simulink model "simulation_rocket"  (R2018a)
settings: Solver=FixedStepAuto  StartTime=0.0  StopTime=200  RelTol=1e-3
undefined symbols (not defined in the file): A_nozzle, area, C_A_0, C_A_Alpha, C_A_Beta, C_Mpitch_alpha, C_Mpitch_q, C_Mroll_0, C_Mroll_p, C_Myaw_beta, C_Myaw_r, C_N_0, C_N_Alpha, C_S_0, C_S_Beta, dot_m, Earth, engine_number, J, l, LF, m, omega_E, omega_J, p_exit, r_gimble, r_init, rotationZ, serial, t_burn, v_exit, WGS84
libraries: aerolibtransform2 x3, aerolibutil x3, instrumentlib x2, aerolibatmos2 x1, aerolibgravity2 x1, sharedutil x1, simulink_extras x1
settings Model: PacingRate=5  ExtModeTrigDuration=2  Creator=hrist  LastModifiedBy=hrist
settings DataIOCC: ExternalInput=[0 0 0 0 0 0]  InitialState=[]  LoadInitialState=on  SaveFormat=StructureWithTime
settings OptimizationCC: EnhancedBackFolding=on  PassReuseOutputArgsAs=Individual arguments  MaxStackSize=64  OptimizeBlockOrder=speed  DifferentSizesBufferReuse=on  OptimizationCustomize=off
settings DebuggingCC: ParameterTunabilityLossMsg=error
settings HardwareCC: ProdBitPerInt=16  ProdBitPerPointer=16  ProdBitPerSizeT=16  ProdBitPerPtrDiffT=16  ProdLargestAtomicFloat=None  ProdWordSize=8  ProdHWDeviceType=Atmel->AVR
settings ModelReferenceCC: PropagateSignalLabelsOutOfModel=off
settings SFSimCC: MATLABDynamicMemAlloc=off
settings RTWCC: SystemTargetFile=ert.tlc  HardwareBoard=Arduino Uno  TLCOptions=-aInlineSetEventsForThisBaseRateFcn=TLC_FALSE -aSuppressMultiTaskScheduler=TLC_FALSE -aRateBasedStepFcn=1  TemplateMakefile=ert_default_tmf  GenerateReport=on  Toolchain=Arduino AVR  BuildConfiguration=Faster Runs  IncludeHyperlinkInReport=on  LaunchReport=on  GenerateTraceInfo=on  GenerateTraceReport=on  GenerateTraceReportSl=on  GenerateTraceReportSf=on  GenerateTraceReportEml=on
settings CodeAppCC: ForceParamTrailComments=on  IgnoreCustomStorageClasses=off  OperatorAnnotations=on  SimulinkDataObjDesc=on  SFDataObjDesc=on  InsertBlockDesc=on
settings ERTTargetCC: SupportContinuousTime=on  SupportVariableSizeSignals=on

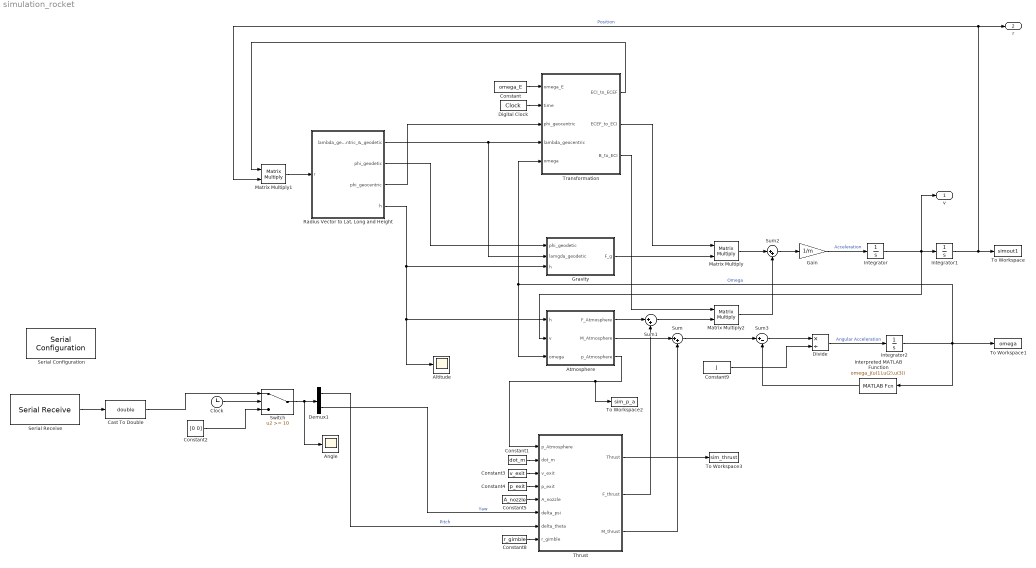
== system simulation_rocket ==
  "Altitude " : Scope
  Angle : Scope
  Atmosphere : Subsystem
  Cast To Double : DataTypeConversion  OutDataTypeStr=double
  Clock : Clock
  Constant : Constant  Value=omega_E
  Constant1 : Constant  Value=dot_m
  Constant2 : Constant  Value=[0 0]  VectorParams1D=off
  Constant3 : Constant  Value=v_exit
  Constant4 : Constant  Value=p_exit
  Constant5 : Constant  Value=A_nozzle
  Constant8 : Constant  Value=r_gimble
  Constant9 : Constant  Value=J  VectorParams1D=off
  Demux1 : Demux  Outputs=2
  Digital Clock : DigitalClock
  Divide : Product  Inputs=*/
  Gain : Gain  Gain=1/m
  Gravity : Subsystem
  Integrator : Integrator  InitialCondition=[600 0 0]
  Integrator1 : Integrator  InitialCondition=r_init
  Integrator2 : Integrator  InitialCondition=[0; 0; 0]
  Interpreted MATLAB Function : MATLABFcn  MATLABFcn=omega_J(u(1),u(2),u(3))
  Matrix Multiply : Product  Multiplication=Matrix(*)
  Matrix Multiply1 : Product  Multiplication=Matrix(*)
  Matrix Multiply2 : Product  Multiplication=Matrix(*)
  "Radius Vector to Lat, Long and Height " : Subsystem
  Serial Configuration : instrumentlib/Serial Configuration  Priority=-200000  ComPortMenu=<Please select a port...>  ComPort=COM6  ObjConstructor=serial('COM6');  BaudRate=115200  DataBits=8  Parity=none  StopBits=1  FlowControl=none  Timeout=10  ByteOrder=LittleEndian
  Serial Receive : instrumentlib/Serial Receive  ComPortMenu=<Please select a port...>  ComPort=COM6  ObjConstructor=serial('COM6');  Header=A  Terminator=LF ('\n')  DataSize="[1  2]"  DataType=single  EnableBlockingMode=on  ActionDataUnavailable=Output last received value  CustomValue=0  SampleTime=0.05
  Sum : Sum  Inputs=|++
  Sum1 : Sum  Inputs=|++
  Sum2 : Sum  Inputs=|++
  Sum3 : Sum  Inputs=|+-
  Switch : Switch  Threshold=10
  Thrust : Subsystem
  To Workspace : ToWorkspace  VariableName=simout1  SaveFormat=Timeseries  SampleTime=-1
  To Workspace1 : ToWorkspace  VariableName=omega  SampleTime=-1
  To Workspace2 : ToWorkspace  VariableName=sim_p_a  SaveFormat=Structure With Time  SampleTime=-1
  To Workspace3 : ToWorkspace  VariableName=sim_thrust  SaveFormat=Structure With Time  SampleTime=-1
  "Transformation " : Subsystem
  v : Outport
  r : Outport  Port=2
  wires:
  Constant/1 -> "Transformation "/1("omega_E ")
  Digital Clock/1 -> "Transformation "/2(time)
  "Radius Vector to Lat, Long and Height "/1("lambda_geocentric_&_geodetic ") -> Gravity/2(lamgda_geodetic), "Transformation "/4(lambda_geocentric)
  "Radius Vector to Lat, Long and Height "/2(phi_geodetic) -> Gravity/1(phi_geodetic)
  "Radius Vector to Lat, Long and Height "/4(h) -> "Altitude "/1, Atmosphere/1(h), Gravity/3(h)
  Atmosphere/3(p_Atmosphere) -> To Workspace2/1, Thrust/1(p_Atmosphere)
  Constant1/1 -> Thrust/2(dot_m)
  Constant3/1 -> Thrust/3(v_exit)
  Constant4/1 -> Thrust/4(p_exit)
  Constant5/1 -> Thrust/5(A_nozzle)
  Constant8/1 -> Thrust/8(r_gimble)
  Atmosphere/2(M_Atmosphere) -> Sum/1
  Thrust/3(M_thrust) -> Sum/2
  Gravity/1(F_g) -> Matrix Multiply/2
  "Transformation "/2(ECEF_to_ECI) -> Matrix Multiply/1
  Atmosphere/1("F_Atmosphere ") -> Sum1/1
  Thrust/2(F_thrust) -> Sum1/2
  Sum1/1 -> Matrix Multiply2/2
  "Transformation "/3(B_to_ECI) -> Matrix Multiply2/1
  Matrix Multiply/1 -> Sum2/1
  Matrix Multiply2/1 -> Sum2/2
  Sum2/1 -> Gain/1
  Gain/1 -> Integrator/1  "Acceleration"
  Integrator1/1 -> r/1, Matrix Multiply1/2, To Workspace/1  "Position"
  Sum/1 -> Sum3/1
  Sum3/1 -> Divide/1
  Constant9/1 -> Divide/2
  Divide/1 -> Integrator2/1  "Angular Acceleration"
  Integrator2/1 -> Interpreted MATLAB Function/1, To Workspace1/1, Atmosphere/3(omega), "Transformation "/5(omega)  "Omega"
  Interpreted MATLAB Function/1 -> Sum3/2
  "Radius Vector to Lat, Long and Height "/3(phi_geocentric) -> "Transformation "/3(phi_geocentric)
  "Transformation "/1(ECI_to_ECEF) -> Matrix Multiply1/1
  Matrix Multiply1/1 -> "Radius Vector to Lat, Long and Height "/1("r ")
  Integrator/1 -> Atmosphere/2(v), v/1, Integrator1/1
  Thrust/1(Thrust) -> To Workspace3/1
  Demux1/1 -> Thrust/7(delta_theta)  "Pitch"
  Demux1/2 -> Thrust/6(delta_psi)  "Yaw"
  Serial Receive/1 -> Cast To Double/1
  Switch/1 -> Angle/1, Demux1/1
  Clock/1 -> Switch/2
  Constant2/1 -> Switch/3
  Cast To Double/1 -> Switch/1

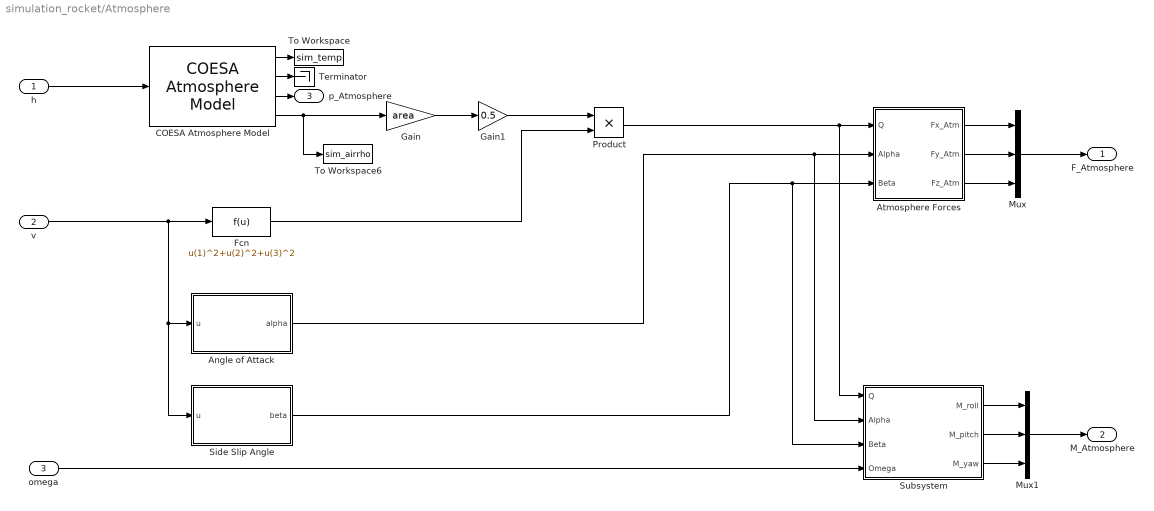
== system simulation_rocket/Atmosphere ==
  h : Inport
  v : Inport  Port=2
  omega : Inport  Port=3
  Angle of Attack : MATLAB Function  TreatAsAtomicUnit=on
  Atmosphere Forces : Subsystem
  COESA Atmosphere Model : aerolibatmos2/COESA Atmosphere Model  units=Metric (MKS)  spec=1976 COESA-extended U.S. Standard Atmosphere  model=Profile  profile_var=High temperature  profile_percent=1%  profile_alt=5 km (16404 ft)  envelope_var=High temperature  envelope_percent=1%  action=Warning
  Fcn : Fcn  Expr=u(1)^2+u(2)^2+u(3)^2
  Gain : Gain  Gain=area
  Gain1 : Gain  Gain=0.5
  Mux : Mux  Inputs=3
  Mux1 : Mux  Inputs=3
  Product : Product
  Side Slip Angle : MATLAB Function  TreatAsAtomicUnit=on
  Subsystem : Subsystem
  Terminator : Terminator
  To Workspace : ToWorkspace  VariableName=sim_temp  SaveFormat=Structure With Time  SampleTime=-1
  To Workspace6 : ToWorkspace  VariableName=sim_airrho  SaveFormat=Structure With Time  SampleTime=-1
  "F_Atmosphere " : Outport
  M_Atmosphere : Outport  Port=2
  p_Atmosphere : Outport  Port=3
  wires:
  COESA Atmosphere Model/2 -> Terminator/1
  h/1 -> COESA Atmosphere Model/1
  v/1 -> Side Slip Angle/1(u), Angle of Attack/1(u), Fcn/1
  COESA Atmosphere Model/4 -> To Workspace6/1, Gain/1
  Gain/1 -> Gain1/1
  Gain1/1 -> Product/1
  Angle of Attack/1(alpha) -> Subsystem/2(Alpha), Atmosphere Forces/2(Alpha)
  Side Slip Angle/1(beta) -> Subsystem/3(Beta), Atmosphere Forces/3(Beta)
  Atmosphere Forces/3(Fz_Atm) -> Mux/3
  Atmosphere Forces/2(Fy_Atm) -> Mux/2
  Atmosphere Forces/1("Fx_Atm ") -> Mux/1
  Mux/1 -> "F_Atmosphere "/1
  Fcn/1 -> Product/2
  omega/1 -> Subsystem/4(Omega)
  Product/1 -> Subsystem/1(Q), Atmosphere Forces/1(Q)
  Subsystem/1(M_roll) -> Mux1/1
  Subsystem/2(M_pitch) -> Mux1/2
  Subsystem/3(M_yaw) -> Mux1/3
  Mux1/1 -> M_Atmosphere/1
  COESA Atmosphere Model/3 -> p_Atmosphere/1
  COESA Atmosphere Model/1 -> To Workspace/1

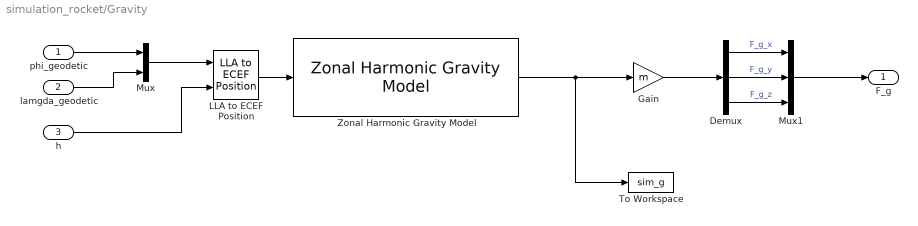
== system simulation_rocket/Gravity ==
  phi_geodetic : Inport
  lamgda_geodetic : Inport  Port=2
  h : Inport  Port=3
  Demux : Demux  Outputs=3
  Gain : Gain  Gain=m
  LLA to ECEF Position : aerolibtransform2/LLA to ECEF Position  units=Metric (MKS)  ptype=Earth (WGS84)  F=1/298.257223563  R=6378137
      settings: SourceProductName=Aerospace Blockset  SourceProductBaseCode=AE
  Mux : Mux  Inputs=2
  Mux1 : Mux  Inputs=3
  To Workspace : ToWorkspace  VariableName=sim_g  SaveFormat=Structure With Time  SampleTime=-1
  Zonal Harmonic Gravity Model : aerolibgravity2/Zonal Harmonic Gravity Model  units=Metric (MKS)  degree=4  action=Warning  ptype=Earth  R=6378136.3  GM=398600441500000  jvalue=[1.0826269e-03 -2.5323000e-06 -1.6204000e-06]
      settings: SourceProductName=Aerospace Blockset  SourceProductBaseCode=AE
  F_g : Outport
  wires:
  LLA to ECEF Position/1 -> Zonal Harmonic Gravity Model/1
  h/1 -> LLA to ECEF Position/2
  Mux/1 -> LLA to ECEF Position/1
  phi_geodetic/1 -> Mux/1
  lamgda_geodetic/1 -> Mux/2
  Zonal Harmonic Gravity Model/1 -> To Workspace/1, Gain/1
  Gain/1 -> Demux/1
  Demux/1 -> Mux1/1  "F_g_x"
  Demux/2 -> Mux1/2  "F_g_y"
  Demux/3 -> Mux1/3  "F_g_z"
  Mux1/1 -> F_g/1

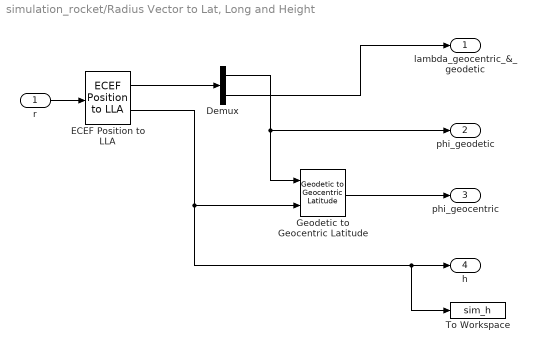
== system simulation_rocket/Radius Vector to Lat, Long and Height  ==
  "r " : Inport
  Demux : Demux  Outputs=2
  ECEF Position to LLA : aerolibtransform2/ECEF Position to LLA  units=Metric (MKS)  ptype=Earth (WGS84)  F=1/298.257223563  R=6378137
      settings: SourceProductName=Aerospace Blockset  SourceProductBaseCode=AE
  Geodetic to Geocentric Latitude : aerolibtransform2/Geodetic to  Geocentric Latitude  units=Metric (MKS)  ptype=Earth (WGS84)  F=1/298.257223563  R=6378137  wraplatitude=on
      settings: SourceProductName=Aerospace Blockset  SourceProductBaseCode=AE
  To Workspace : ToWorkspace  VariableName=sim_h  SaveFormat=Structure With Time  SampleTime=-1
  "lambda_geocentric_&_geodetic " : Outport
  phi_geodetic : Outport  Port=2
  phi_geocentric : Outport  Port=3
  h : Outport  Port=4
  wires:
  "r "/1 -> ECEF Position to LLA/1
  ECEF Position to LLA/1 -> Demux/1
  ECEF Position to LLA/2 -> To Workspace/1, h/1, Geodetic to Geocentric Latitude/2
  Demux/1 -> phi_geodetic/1, Geodetic to Geocentric Latitude/1
  Demux/2 -> "lambda_geocentric_&_geodetic "/1
  Geodetic to Geocentric Latitude/1 -> phi_geocentric/1

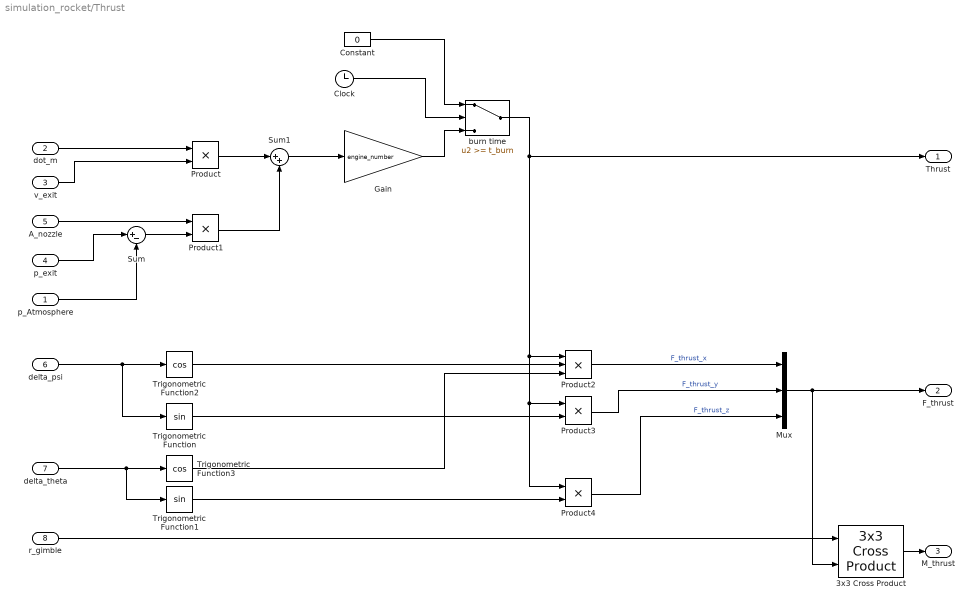
== system simulation_rocket/Thrust ==
  p_Atmosphere : Inport
  dot_m : Inport  Port=2
  v_exit : Inport  Port=3
  p_exit : Inport  Port=4
  A_nozzle : Inport  Port=5
  delta_psi : Inport  Port=6
  delta_theta : Inport  Port=7
  r_gimble : Inport  Port=8
  3x3 Cross Product : sharedutil/3x3 Cross Product  aMode=aMode
      settings: SourceProductBaseCode=AE
  Clock : Clock
  Constant : Constant  Value=0
  Gain : Gain  Gain=engine_number
  Mux : Mux  Inputs=3
  Product{,1,3..4} (4 alike) : Product
  Product2 : Product  Inputs=3
  Sum : Sum  Inputs=|+-
  Sum1 : Sum  Inputs=|++
  Trigonometric Function : Trigonometry
  Trigonometric Function1 : Trigonometry
  Trigonometric Function2 : Trigonometry  Operator=cos
  Trigonometric Function3 : Trigonometry  Operator=cos
  burn time : Switch  Threshold=t_burn
  Thrust : Outport
  F_thrust : Outport  Port=2
  M_thrust : Outport  Port=3
  wires:
  dot_m/1 -> Product/1
  v_exit/1 -> Product/2
  A_nozzle/1 -> Product1/1
  Sum/1 -> Product1/2
  p_exit/1 -> Sum/1
  p_Atmosphere/1 -> Sum/2
  Product/1 -> Sum1/1
  Product1/1 -> Sum1/2
  Sum1/1 -> Gain/1
  delta_psi/1 -> Trigonometric Function/1, Trigonometric Function2/1
  delta_theta/1 -> Trigonometric Function1/1, Trigonometric Function3/1
  Trigonometric Function2/1 -> Product2/2
  Trigonometric Function3/1 -> Product2/3
  Trigonometric Function/1 -> Product3/2
  Trigonometric Function1/1 -> Product4/2
  Product2/1 -> Mux/1  "F_thrust_x"
  Product3/1 -> Mux/2  "F_thrust_y"
  Product4/1 -> Mux/3  "F_thrust_z"
  Mux/1 -> 3x3 Cross Product/2, F_thrust/1
  r_gimble/1 -> 3x3 Cross Product/1
  3x3 Cross Product/1 -> M_thrust/1
  burn time/1 -> Thrust/1, Product4/1, Product3/1, Product2/1
  Constant/1 -> burn time/1
  Clock/1 -> burn time/2
  Gain/1 -> burn time/3

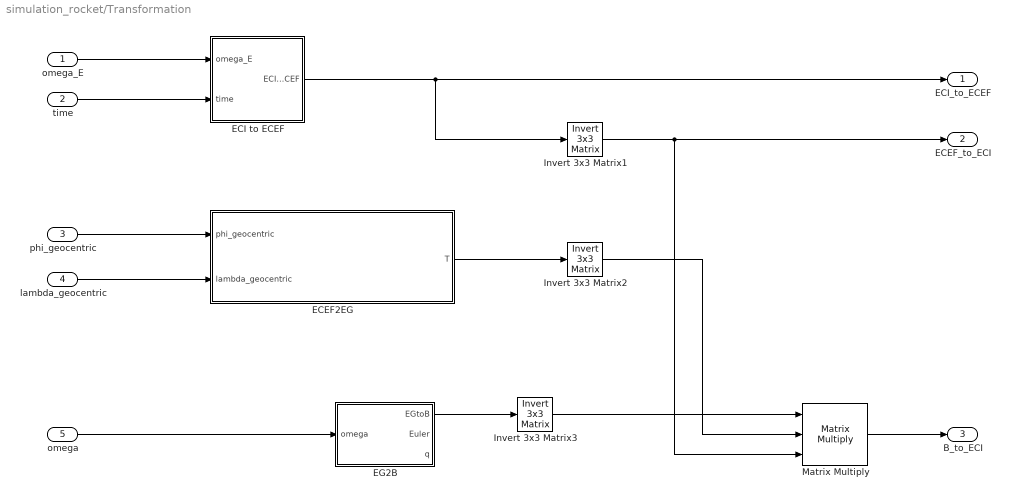
== system simulation_rocket/Transformation  ==
  "omega_E " : Inport
  time : Inport  Port=2
  phi_geocentric : Inport  Port=3
  lambda_geocentric : Inport  Port=4
  omega : Inport  Port=5
  ECEF2EG : MATLAB Function  TreatAsAtomicUnit=on
  ECI to ECEF : Subsystem
  EG2B : Subsystem
  Invert 3x3 Matrix1 : aerolibutil/Invert  3x3 Matrix
  Invert 3x3 Matrix2 : aerolibutil/Invert  3x3 Matrix
  Invert 3x3 Matrix3 : aerolibutil/Invert  3x3 Matrix
  Matrix Multiply : Product  Inputs=3  Multiplication=Matrix(*)
  ECI_to_ECEF : Outport
  ECEF_to_ECI : Outport  Port=2
  B_to_ECI : Outport  Port=3
  wires:
  "omega_E "/1 -> ECI to ECEF/1(omega_E)
  time/1 -> ECI to ECEF/2(time)
  phi_geocentric/1 -> ECEF2EG/1(phi_geocentric)
  lambda_geocentric/1 -> ECEF2EG/2(lambda_geocentric)
  ECEF2EG/1(T) -> Invert 3x3 Matrix2/1
  Matrix Multiply/1 -> B_to_ECI/1
  ECI to ECEF/1(ECI_to_ECEF) -> ECI_to_ECEF/1, Invert 3x3 Matrix1/1
  Invert 3x3 Matrix2/1 -> Matrix Multiply/2
  Invert 3x3 Matrix1/1 -> ECEF_to_ECI/1, Matrix Multiply/3
  omega/1 -> EG2B/1(omega)
  Invert 3x3 Matrix3/1 -> Matrix Multiply/1
  EG2B/1(EGtoB) -> Invert 3x3 Matrix3/1

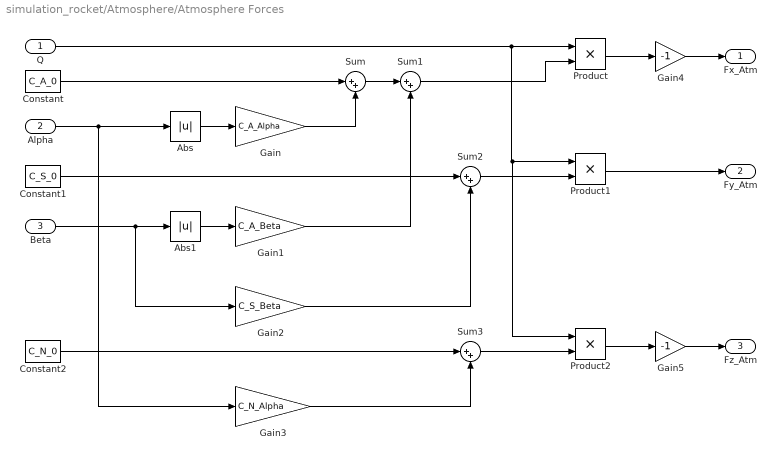
== system simulation_rocket/Atmosphere/Atmosphere Forces ==
  Q : Inport
  Alpha : Inport  Port=2
  Beta : Inport  Port=3
  Abs : Abs
  Abs1 : Abs
  Constant : Constant  Value=C_A_0
  Constant1 : Constant  Value=C_S_0
  Constant2 : Constant  Value=C_N_0
  Gain : Gain  Gain=C_A_Alpha
  Gain1 : Gain  Gain=C_A_Beta
  Gain2 : Gain  Gain=C_S_Beta
  Gain3 : Gain  Gain=C_N_Alpha
  Gain4 : Gain  Gain=-1
  Gain5 : Gain  Gain=-1
  Product : Product
  Product1 : Product
  Product2 : Product
  Sum{,1..3} (4 alike) : Sum  Inputs=|++
  "Fx_Atm " : Outport
  Fy_Atm : Outport  Port=2
  Fz_Atm : Outport  Port=3
  wires:
  Constant/1 -> Sum/1
  Alpha/1 -> Gain3/1, Abs/1
  Abs/1 -> Gain/1
  Gain/1 -> Sum/2
  Beta/1 -> Gain2/1, Abs1/1
  Abs1/1 -> Gain1/1
  Sum/1 -> Sum1/1
  Gain1/1 -> Sum1/2
  Sum1/1 -> Product/2
  Constant1/1 -> Sum2/1
  Gain2/1 -> Sum2/2
  Sum2/1 -> Product1/2
  Constant2/1 -> Sum3/1
  Gain3/1 -> Sum3/2
  Sum3/1 -> Product2/2
  Q/1 -> Product2/1, Product1/1, Product/1
  Product1/1 -> Fy_Atm/1
  Product/1 -> Gain4/1
  Gain4/1 -> "Fx_Atm "/1
  Product2/1 -> Gain5/1
  Gain5/1 -> Fz_Atm/1

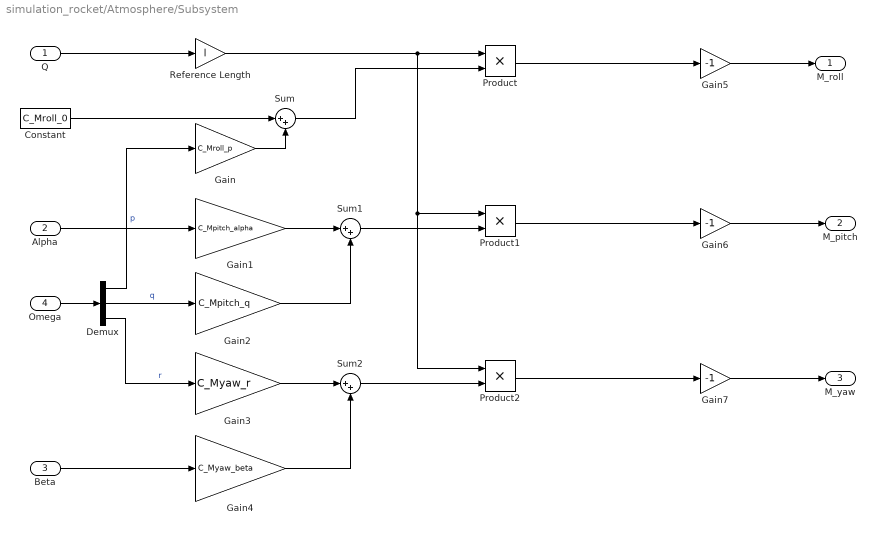
== system simulation_rocket/Atmosphere/Subsystem ==
  Q : Inport
  Alpha : Inport  Port=2
  Beta : Inport  Port=3
  Omega : Inport  Port=4
  Constant : Constant  Value=C_Mroll_0
  Demux : Demux  Outputs=3
  Gain : Gain  Gain=C_Mroll_p
  Gain1 : Gain  Gain=C_Mpitch_alpha
  Gain2 : Gain  Gain=C_Mpitch_q
  Gain3 : Gain  Gain=C_Myaw_r
  Gain4 : Gain  Gain=C_Myaw_beta
  Gain5 : Gain  Gain=-1
  Gain6 : Gain  Gain=-1
  Gain7 : Gain  Gain=-1
  Product : Product
  Product1 : Product
  Product2 : Product
  Reference Length : Gain  Gain=l
  Sum : Sum  Inputs=|++
  Sum1 : Sum  Inputs=|++
  Sum2 : Sum  Inputs=|++
  M_roll : Outport
  M_pitch : Outport  Port=2
  M_yaw : Outport  Port=3
  wires:
  Q/1 -> Reference Length/1
  Omega/1 -> Demux/1
  Demux/1 -> Gain/1  "p"
  Constant/1 -> Sum/1
  Gain/1 -> Sum/2
  Reference Length/1 -> Product2/1, Product1/1, Product/1
  Sum/1 -> Product/2
  Alpha/1 -> Gain1/1
  Demux/2 -> Gain2/1  "q"
  Gain1/1 -> Sum1/1
  Gain2/1 -> Sum1/2
  Sum1/1 -> Product1/2
  Demux/3 -> Gain3/1  "r"
  Beta/1 -> Gain4/1
  Gain3/1 -> Sum2/1
  Gain4/1 -> Sum2/2
  Sum2/1 -> Product2/2
  Product2/1 -> Gain7/1
  Product1/1 -> Gain6/1
  Product/1 -> Gain5/1
  Gain5/1 -> M_roll/1
  Gain6/1 -> M_pitch/1
  Gain7/1 -> M_yaw/1

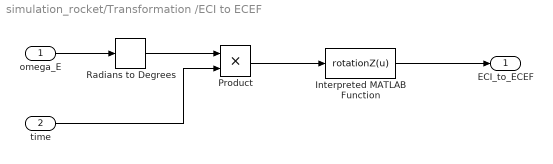
== system simulation_rocket/Transformation /ECI to ECEF ==
  omega_E : Inport
  time : Inport  Port=2
  Interpreted MATLAB Function : MATLABFcn  MATLABFcn=rotationZ(u)  Output1D=off
  Product : Product
  Radians to Degrees : simulink_extras/Transformations/Radians to Degrees
  ECI_to_ECEF : Outport
  wires:
  omega_E/1 -> Radians to Degrees/1
  Radians to Degrees/1 -> Product/1
  time/1 -> Product/2
  Product/1 -> Interpreted MATLAB Function/1
  Interpreted MATLAB Function/1 -> ECI_to_ECEF/1

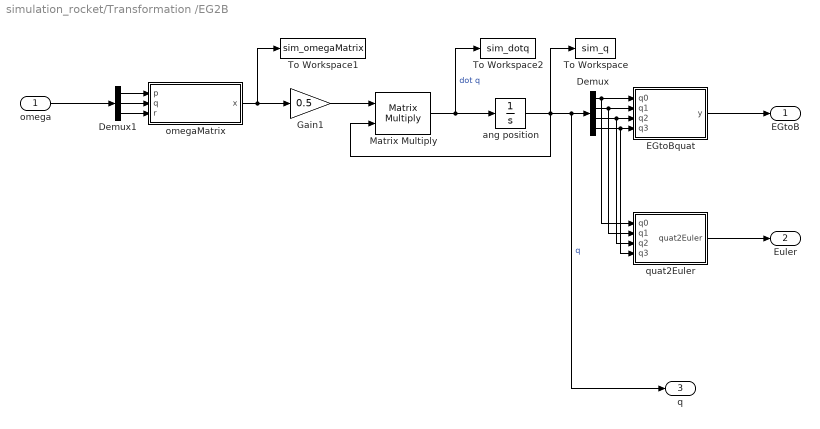
== system simulation_rocket/Transformation /EG2B ==
  omega : Inport
  Demux : Demux
  Demux1 : Demux  Outputs=3
  EGtoBquat : MATLAB Function  TreatAsAtomicUnit=on
  Gain1 : Gain  Gain=0.5
  Matrix Multiply : Product  Multiplication=Matrix(*)
  To Workspace : ToWorkspace  VariableName=sim_q  SaveFormat=Structure With Time  SampleTime=-1
  To Workspace1 : ToWorkspace  VariableName=sim_omegaMatrix  SaveFormat=Structure With Time  SampleTime=-1
  To Workspace2 : ToWorkspace  VariableName=sim_dotq  SaveFormat=Structure With Time  SampleTime=-1
  ang position : Integrator  InitialCondition=[1; 0; 0; 0]
  omegaMatrix : MATLAB Function  TreatAsAtomicUnit=on
  quat2Euler : MATLAB Function  TreatAsAtomicUnit=on
  EGtoB : Outport
  Euler : Outport  Port=2
  q : Outport  Port=3
  wires:
  ang position/1 -> To Workspace/1, q/1, Demux/1, Matrix Multiply/2  "q"
  Demux1/3 -> omegaMatrix/3(r)
  Matrix Multiply/1 -> To Workspace2/1, ang position/1  "dot q"
  Demux1/2 -> omegaMatrix/2(q)
  Demux/3 -> quat2Euler/3(q2), EGtoBquat/3(q2)
  omegaMatrix/1(x) -> To Workspace1/1, Gain1/1
  Demux/1 -> quat2Euler/1(q0), EGtoBquat/1(q0)
  Demux1/1 -> omegaMatrix/1(p)
  Gain1/1 -> Matrix Multiply/1
  Demux/2 -> quat2Euler/2(q1), EGtoBquat/2(q1)
  Demux/4 -> quat2Euler/4(q3), EGtoBquat/4(q3)
  omega/1 -> Demux1/1
  EGtoBquat/1(y) -> EGtoB/1
  quat2Euler/1(quat2Euler) -> Euler/1

== matlab function simulation_rocket/Transformation /ECEF2EG ==
  data: phi_geocentric input; T output; lambda_geocentric input
%% Transformation matrix function ECEF to EG

function T  = ECEF_to_EG(phi_geocentric,lambda_geocentric)

    T=rotationY(-phi_geocentric)*rotationZ(lambda_geocentric);
    
end

== matlab function simulation_rocket/Atmosphere/Angle of Attack ==
  data: u input; alpha output
function alpha = Alpha(u)
    alpha = 0;
    if (u(1) ~= 0)
        alpha = atan2d(u(3), u(1));
    end

end

== matlab function simulation_rocket/Atmosphere/Side Slip Angle ==
  data: u input; beta output
function beta = Beta(u)
    beta=0;
    if (u(1)~=0)
        beta=-atan2d(u(2),u(1));
    end
    
    if abs(beta) < 1e-5
        beta = 0;
    end
end

== matlab function simulation_rocket/Transformation /EG2B/EGtoBquat ==
  data: q0 input; y output; q1 input; q2 input; q3 input
%% Transformation quaternion matrix from EG to B
function y = u(q0, q1, q2, q3)
    y = [q0^2 + q1^2 - q2^2 - q3^2, 2*q1*q2 - 2*q0*q3,          2*q0*q2 + 2*q1*q3;
         2*q0*q3 + 2*q1*q2,         q0^2 - q1^2 + q2^2 - q3^2,  2*q2*q3 - 2*q0*q1;
         2*q1*q3 - 2*q0*q2,         2*q0*q1 + 2*q2*q3,          q0^2 - q1^2 - q2^2 + q3^2];
end

== matlab function simulation_rocket/Transformation /EG2B/omegaMatrix ==
  data: p input; x output; q input; r input
%% Creates matrix from equation 2.13
function x  = omegaMatrix(p, q, r)
    x = [0 -p -q -r;
         p 0 r -q;
         q -r 0 p;
         r q -p 0];
end

== matlab function simulation_rocket/Transformation /EG2B/quat2Euler ==
  data: q0 input; quat2Euler output; q1 input; q2 input; q3 input
%% Returns Euler angles from quaternions.
function quat2Euler = u(q0, q1, q2, q3)
    newphi = atan(2*(q2*q3+q0*q1)/(q0^2 - q1^2 - q2^2 + q3^2));
    newtheta = asin(2*(q0*q2 - q1*q3));
    newpsi = atan(2*(q1*q2+q0*q3)/(q0^2 + q1^2 - q2^2 - q3^2));
    
    quat2Euler = [newphi; newtheta; newpsi];
end
